simulink model "Frequency_squarechirp"  (R2021b)
settings: Solver=ode4  StartTime=0.0  StopTime=310  FixedStep=0.02  RelTol=1e-3
settings Model: Creator=Tara.Aryal  LastModifiedBy=Tara.Aryal
settings RTWCC: GenCodeOnly=on  PackageGeneratedCodeAndArtifacts=on  PackageName=squarecode.zip
settings CodeAppCC: MaxIdLength=50
settings GRTTargetCC: CombineOutputUpdateFcns=off

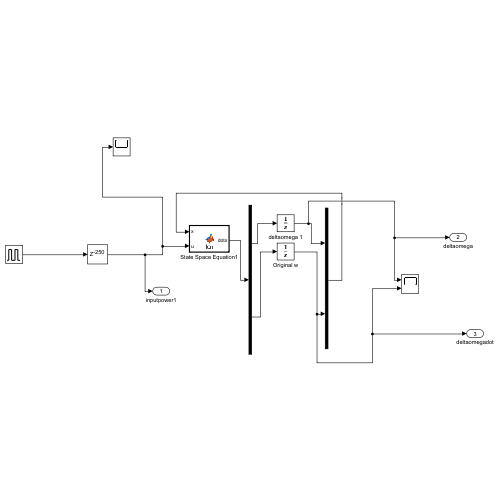
[thumbnail: Simulink's stored preview of the top-level diagram]
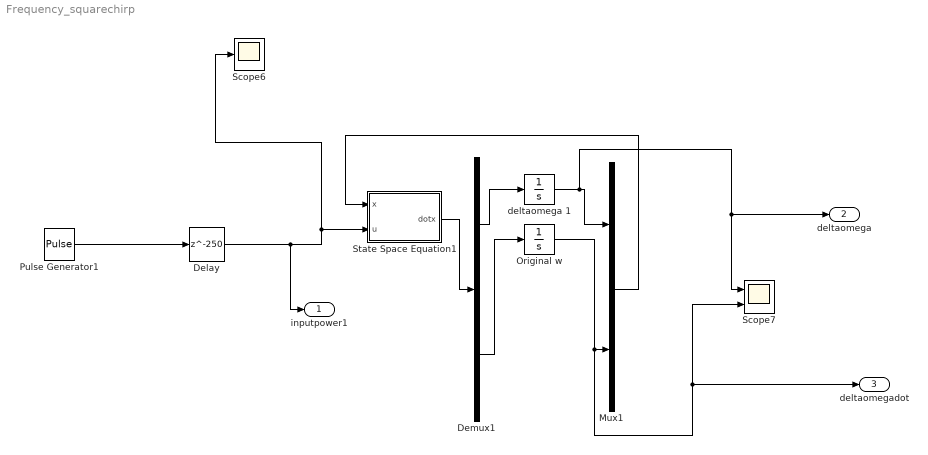
== system Frequency_squarechirp ==
  Delay : Delay  DelayLength=250
  Demux1 : Demux  Outputs=2
  Mux1 : Mux  Inputs=2
  Original w : Integrator
  Pulse Generator1 : DiscretePulseGenerator  PulseType=Time based  Amplitude=0.1  Period=1  PulseWidth=50
  Scope6 : Scope
  Scope7 : Scope  NumInputPorts=2
  State Space Equation1 : MATLAB Function  TreatAsAtomicUnit=on
  deltaomega 1 : Integrator
  inputpower1 : Outport
  deltaomega : Outport  Port=2
  deltaomegadot : Outport  Port=3
  wires:
  Demux1/1 -> deltaomega 1/1
  Delay/1 -> inputpower1/1, Scope6/1, State Space Equation1/2(u)
  Mux1/1 -> State Space Equation1/1(x)
  deltaomega 1/1 -> deltaomega/1, Scope7/1, Mux1/1
  Demux1/2 -> Original w/1
  Original w/1 -> Mux1/2, Scope7/2, deltaomegadot/1
  State Space Equation1/1(dotx) -> Demux1/1
  Pulse Generator1/1 -> Delay/1

== matlab function Frequency_squarechirp/State Space Equation1 ==
  data: x input; u input; dotx output
function dotx  = fcn(x, u)
D = 1.5/100;
M = 3.0;
    Tg = 0.2;
    Rp = 0.05;
    Ki=2;
    dotx = zeros(2, 1);
    %x1 = x(1);
    x1 = x(1);
    x2=x(2);
    dotx = [x2;-(D/(M*Tg)+1/(Rp*M*Tg))*x1-(D/M+1/Tg)*x2-1/(M*Tg)*u];
